simulink model "dis_nonlin"  (R2020b)
settings: Solver=VariableStepAuto  StartTime=0.0  StopTime=50.0  RelTol=1e-3
values from neighbouring files (symbols this model uses):
  alpha = 0.95    [main.m]
  amp = 0.3    [main.m]
  Ts = 0.15    [main.m]
  u_equ = 0.16    [main.m]
  x_equ = [0.2; 0]    [main.m]
settings Model: Creator=soren  LastModifiedBy=soren

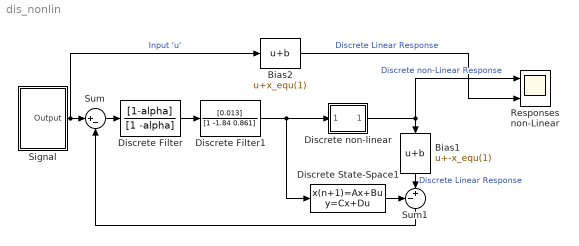
== system dis_nonlin ==
  Bias1 : Bias  Bias=-x_equ(1)
  Bias2 : Bias  Bias=x_equ(1)
  Discrete Filter : DiscreteFilter  Numerator=[1-alpha]  Denominator=[1 -alpha]
  Discrete Filter1 : DiscreteFilter  Numerator=[0.013]  Denominator=[1 -1.84 0.861]
  Discrete State-Space1 : DiscreteStateSpace  A=[1 Ts;-3/4*Ts 1-Ts]  B=[0; 1.25*Ts]  C=[1, 0]  D=0  SampleTime=Ts
  Discrete non-linear : Subsystem
  Responses non-Linear : Scope  NumInputPorts=2
  Signal : Subsystem
  Sum : Sum  Inputs=|+-
  Sum1 : Sum  Inputs=-+|
  wires:
  Sum/1 -> Discrete Filter/1
  Discrete State-Space1/1 -> Sum1/1
  Sum1/1 -> Sum/2
  Signal/1(Output) -> Bias2/1, Sum/1  "Input 'u'"
  Discrete Filter/1 -> Discrete Filter1/1
  Discrete Filter1/1 -> Discrete non-linear/1(Input1), Discrete State-Space1/1
  Discrete non-linear/1(Output) -> Responses non-Linear/1, Bias1/1  "Discrete non-Linear Response"
  Bias1/1 -> Sum1/2  "Discrete Linear Response"
  Bias2/1 -> Responses non-Linear/2  "Discrete Linear Response"

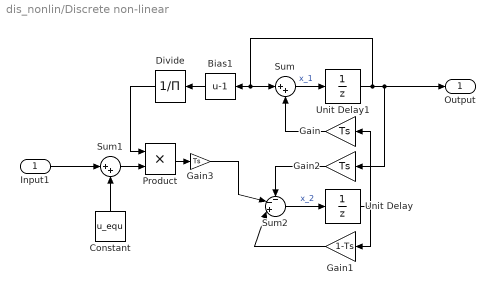
== system dis_nonlin/Discrete non-linear ==
  Input1 : Inport  SampleTime=Ts
  Bias1 : Bias  Bias=-1
  Constant : Constant  Value=u_equ
  Divide : Product  Inputs=/
  Gain : Gain  Gain=Ts
  Gain1 : Gain  Gain=1-Ts
  Gain2 : Gain  Gain=Ts
  Gain3 : Gain  Gain=Ts
  Product : Product
  Sum : Sum  Inputs=|++
  Sum1 : Sum  Inputs=|++
  Sum2 : Sum  Inputs=--+|
  Unit Delay : UnitDelay  SampleTime=-1  HasFrameUpgradeWarning=on
  Unit Delay1 : UnitDelay  InitialCondition=x_equ(1)  SampleTime=-1  HasFrameUpgradeWarning=on
  Output : Outport  SampleTime=Ts
  wires:
  Constant/1 -> Sum1/2
  Unit Delay1/1 -> Bias1/1, Sum/1, Gain2/1, Output/1
  Input1/1 -> Sum1/1
  Sum/1 -> Unit Delay1/1  "x_1"
  Sum1/1 -> Product/2
  Bias1/1 -> Divide/1
  Sum2/1 -> Unit Delay/1  "x_2"
  Divide/1 -> Product/1
  Unit Delay/1 -> Gain1/1, Gain/1
  Gain/1 -> Sum/2
  Gain1/1 -> Sum2/3
  Gain2/1 -> Sum2/1
  Product/1 -> Gain3/1
  Gain3/1 -> Sum2/2

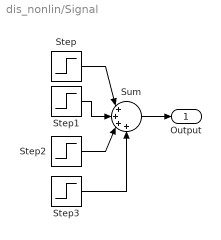
== system dis_nonlin/Signal ==
  Step : Step  Time=10  After=0.2*amp  SampleTime=0
  Step1 : Step  Time=20  After=-0.2*amp  SampleTime=0
  Step2 : Step  Time=30  After=-0.2*amp  SampleTime=0
  Step3 : Step  Time=40  After=0.2*amp  SampleTime=0
  Sum : Sum  Inputs=|++++
  Output : Outport
  wires:
  Sum/1 -> Output/1
  Step2/1 -> Sum/3
  Step/1 -> Sum/1
  Step1/1 -> Sum/2
  Step3/1 -> Sum/4
